simulink model "modelo"  (R2018b)
settings: Solver=VariableStepAuto  StartTime=0.0  StopTime=5  RelTol=1e-3
values from neighbouring files (symbols this model uses):
  A = [0      1              0           0 ... (first row only)    [intento.m]    (also in prueba.m; task.m = [             0, 1, 0,                   0; task_LQR.m = [             0, 1, 0,                   0; task_PID.m = [             0, 1, 0,                   0)
  B = [     0 ... (first row only)    [intento.m]    (also in prueba.m; task.m = [0; -M*L/p; 0; (I+M*L^2)/p]; task_LQR.m = [0; -M*L/p; 0; (I+M*L^2)/p]; task_PID.m = [0; -M*L/p; 0; (I+M*L^2)/p])
  Kd = 1    [intento.m]    (also in task.m = 0.005; task_PID.m = 0.005)
  Ki = 1    [intento.m]    (also in task.m = 0.5; task_PID.m = 14)
  Kp = 1    [intento.m]    (also in task.m = 1.5; task_PID.m = 0.4)
  x0 = [0.2; 0; 0; 0]    [intento.m]    (also in prueba.m = [0; 0; 0.2; 0]; task.m; task_LQR.m; task_PID.m)
undefined symbols (not defined in the file or in its folder): K1, K2, K3, K4
libraries: simulink x1
settings Model: Creator=vuvux  LastModifiedBy=vuvux

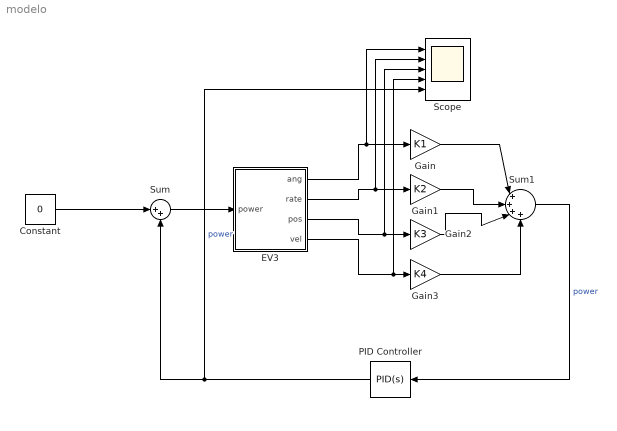
== system modelo ==
  Constant : Constant  Value=0
  "EV3 " : Subsystem
  Gain : Gain  Gain=K1
  Gain1 : Gain  Gain=K2
  Gain2 : Gain  Gain=K3
  Gain3 : Gain  Gain=K4
  PID Controller : simulink/Continuous/PID Controller  Controller=PID  Form=Parallel  TimeDomain=Continuous-time  SampleTime=-1  IntegratorMethod=Forward Euler  FilterMethod=Forward Euler  ControllerParametersSource=internal  P=Kp  I=Ki  D=Kd  UseFilter=on  N=6423.35488320633  TunerSelectOption=Transfer Function Based (PID Tuner App)  InitialConditionSource=internal  InitialConditionForIntegrator=0  InitialConditionForFilter=0  DifferentiatorICPrevScaledInput=0  ExternalReset=none  TrackingMode=off  Kt=1  LimitOutput=off  UpperSaturationLimit=inf  LowerSaturationLimit=-inf  LinearizeAsGain=on  AntiWindupMode=none  Kb=1  POutMin=[]  POutMax=[]  IOutMin=[]  IOutMax=[]  DOutMin=[]  DOutMax=[]  NOutMin=[]  NOutMax=[]  SumOutMin=[]  SumOutMax=[]  SaturationOutMin=[]  SaturationOutMax=[]  PParamMin=[]  PParamMax=[]  IParamMin=[]  IParamMax=[]  DParamMin=[]  DParamMax=[]  NParamMin=[]  NParamMax=[]  KbParamMin=[]  KbParamMax=[]  KtParamMin=[]  KtParamMax=[]  KbOutMin=[]  KbOutMax=[]  KtOutMin=[]  KtOutMax=[]  IntegratorOutMin=[]  IntegratorOutMax=[]  FilterOutMin=[]  FilterOutMax=[]  SumI1OutMin=[]  SumI1OutMax=[]  SumI2OutMin=[]  SumI2OutMax=[]  SumI3OutMin=[]  SumI3OutMax=[]  SumI4OutMin=[]  SumI4OutMax=[]  SumDOutMin=[]  SumDOutMax=[]  DifferentiatorOutMin=[]  DifferentiatorOutMax=[]  FilterDiffOutCoefMin=[]  FilterDiffOutCoefMax=[]  ReciprocalOutMin=[]  ReciprocalOutMax=[]  SumDenOutMin=[]  SumDenOutMax=[]  SumNumOutMin=[]  SumNumOutMax=[]  DivideOutMin=[]  DivideOutMax=[]  IntegratorContinuousStateAttributes=''  IntegratorStateMustResolveToSignalObject=off  IntegratorRTWStateStorageClass=Auto  FilterContinuousStateAttributes=''  FilterStateMustResolveToSignalObject=off  FilterRTWStateStorageClass=Auto  ParallelPVariant=InternalParameters  IdealPVariant=Disabled  IVariant=InternalParameters  DVariant=InternalParameters  IntegratorVariant=Continuous  SatVariant=Disabled  AWVariant=Passthrough  PCopyVariant=Disabled  TRVariant=Disabled  FdbkBlocksVariant=Forward  IdealPFdbkVariant=Disabled  SatFdbkVariant=Disabled  DerivativeFilterVariant=ContFilter  NVariant=InternalParameters  NCopyVariant=Disabled  FilterICVariant=InternalICsFilter  IntegratorICVariant=InternalICs  ExternalResetVariant=Disabled  TRSumVariant=Passthrough  SumFdbkVariant=Disabled  SumVariant=Sum_PID
  Scope : Scope  NumInputPorts=5
  Sum : Sum  Inputs=|++
  Sum1 : Sum  Inputs=|++++
  wires:
  Constant/1 -> Sum/1
  Sum1/1 -> PID Controller/1  "power"
  Sum/1 -> "EV3 "/1(power)
  Gain/1 -> Sum1/1
  Gain1/1 -> Sum1/2
  Gain2/1 -> Sum1/3
  Gain3/1 -> Sum1/4
  "EV3 "/1(ang) -> Scope/1, Gain/1
  "EV3 "/2(rate) -> Gain1/1, Scope/2
  "EV3 "/3(pos) -> Gain2/1, Scope/3
  "EV3 "/4(vel) -> Scope/4, Gain3/1
  PID Controller/1 -> Scope/5, Sum/2  "power"

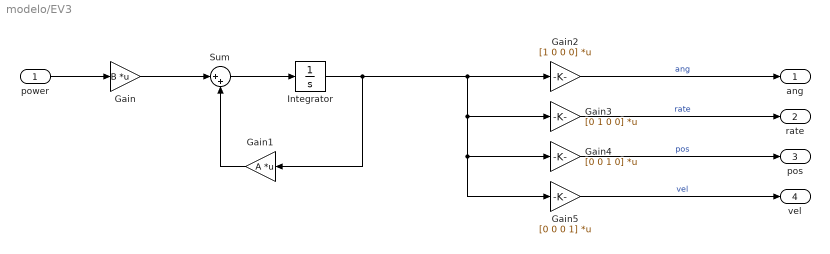
== system modelo/EV3  ==
  power : Inport
  Gain : Gain  Gain=B  Multiplication=Matrix(K*u)
  Gain1 : Gain  Gain=A  Multiplication=Matrix(K*u)
  Gain2 : Gain  Gain=[1 0 0 0]  Multiplication=Matrix(K*u)
  Gain3 : Gain  Gain=[0 1 0 0]  Multiplication=Matrix(K*u)
  Gain4 : Gain  Gain=[0 0 1 0]  Multiplication=Matrix(K*u)
  Gain5 : Gain  Gain=[0 0 0 1]  Multiplication=Matrix(K*u)
  Integrator : Integrator  InitialCondition=x0
  Sum : Sum  Inputs=|++
  ang : Outport
  rate : Outport  Port=2
  pos : Outport  Port=3
  vel : Outport  Port=4
  wires:
  Gain1/1 -> Sum/2
  Gain/1 -> Sum/1
  Sum/1 -> Integrator/1
  Integrator/1 -> Gain1/1, Gain2/1, Gain3/1, Gain4/1, Gain5/1
  power/1 -> Gain/1
  Gain4/1 -> pos/1  "pos"
  Gain3/1 -> rate/1  "rate"
  Gain5/1 -> vel/1  "vel"
  Gain2/1 -> ang/1  "ang"
